simulink model "MixailFiltr_02m"  (R2017a)
settings: Solver=FixedStepAuto  StartTime=0.0  StopTime=40.67  FixedStep=0.01  RelTol=1e-3
InitFcn:
  | mSig(1:10) = 0;
  | mSig(11:35) = 20;
  | mSig(36:40) = 0;
  | t01=0.01.*(1:length(mSig));
  | tImpuls = zeros(length(mSig), 2);
  | tImpuls(:,2) = mSig;
  | tImpuls(:,1) = t01;
libraries: MyEma x1
settings Model: Creator=alexandr.lanin  LastModifiedBy=alexandr.lanin
settings SolverCC: MaxConsecutiveMinStep=auto

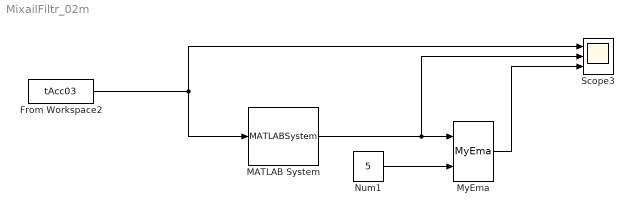
== system MixailFiltr_02m ==
  From Workspace2 : FromWorkspace  VariableName=tAcc03  SampleTime=0.01
  MATLAB System : MATLABSystem  System=MixFiltrSig  SimulateUsing=Code generation
      mask Type: MixFiltrSig
      mask Display:
      | disp('MixFiltrSig');
      | port_label('input',1,'u');
      | port_label('output',1,'y');
  MyEma : MyEma/MyEma
  Num1 : Constant  Value=5
  Scope3 : Scope  NumInputPorts=3
  wires:
  MATLAB System/1 -> MyEma/1, Scope3/2
  MyEma/1 -> Scope3/3
  Num1/1 -> MyEma/2
  From Workspace2/1 -> MATLAB System/1, Scope3/1
